simulink model "model_in_the_loop"  (R2017a)
settings: Solver=VariableStepAuto  StartTime=0.0  StopTime=10.0  RelTol=1e-3
values from neighbouring files (symbols this model uses):
  a = 31    [fun_h1.m]    (also in fun_h2.m; fun_h3.m; identyfikacja_sqrt_h1.m; lqr_indentyfikacja.m)
  b = 46.5    [fun_h2.m]    (also in identyfikacja_sqrt_h1.m = [(C1_0+delta_C1_0); (C1_0-delta_C1_0); (D1_0+delta_D1_0); (-; identyfikacja_sqrt_h2.m = [(C2_0+delta_C2_0); (C2_0-delta_C2_0); (D2_0+delta_D2_0); (-; identyfikacja_sqrt_h3.m = [(C3_0+delta_C3_0); (C3_0-delta_C3_0); (D3_0+delta_D3_0); (-; lqr_indentyfikacja.m)
  c = 10    [fun_h2.m]    (also in lqr_indentyfikacja.m; run_model.m)
  C1max = 36.9    [lqr_indentyfikacja.m]    (also in run_model.m)
  C2max = 33.91    [lqr_indentyfikacja.m]    (also in run_model.m)
  C3max = 36    [lqr_indentyfikacja.m]    (also in run_model.m)
  D1 = teta(2)    [fun_h1.m]    (also in lqr_indentyfikacja.m = 3.5673; run_model.m = 3.5673)
  D2 = teta(2)    [fun_h2.m]    (also in lqr_indentyfikacja.m = 2.8498; run_model.m = 2.8498)
  D3 = teta(2)    [fun_h3.m]    (also in lqr_indentyfikacja.m = 2.882; run_model.m = 2.882)
  gC1 = 1    [lqr_indentyfikacja.m]    (also in run_model.m)
  gC2 = 1    [lqr_indentyfikacja.m]    (also in run_model.m)
  gC3 = 1    [lqr_indentyfikacja.m]    (also in run_model.m)
  H10 = teta(4)    [fun_h1.m]    (also in lqr_indentyfikacja.m = 11.9703; run_model.m = 11.9703)
  H1OUT = ((C2*(r+D2)^p2)/C1)^2    (= 11.9703137378)    [lqr_indentyfikacja.m]
  H20 = teta(4)    [fun_h2.m]    (also in lqr_indentyfikacja.m = 15; run_model.m = 15)
  H2OUT = r    (= 15)    [lqr_indentyfikacja.m]
  H30 = teta(4)    [fun_h3.m]    (also in lqr_indentyfikacja.m = 12.5763; run_model.m = 12.5763)
  H3OUT = ((C2*(r+D2)^p2)/C3)^2    (= 12.5763108708)    [lqr_indentyfikacja.m]
  Hmax = 40    [lqr_indentyfikacja.m]    (also in run_model.m)
  p1 = teta(3)    [fun_h1.m]    (also in lqr_indentyfikacja.m = 0.41; run_model.m = 0.41)
  p2 = teta(3)    [fun_h2.m]    (also in lqr_indentyfikacja.m = 0.46; run_model.m = 0.46)
  p3 = teta(3)    [fun_h3.m]    (also in lqr_indentyfikacja.m = 0.37; run_model.m = 0.37)
  R = 20    [lqr_indentyfikacja.m]    (also in run_model.m = 39)
  w = 5    [fun_h1.m]    (also in fun_h2.m; fun_h3.m; lqr_indentyfikacja.m; run_model.m)
undefined symbols (not defined in the file or in its folder): K
settings Model: Creator=thepi  LastModifiedBy=thepi

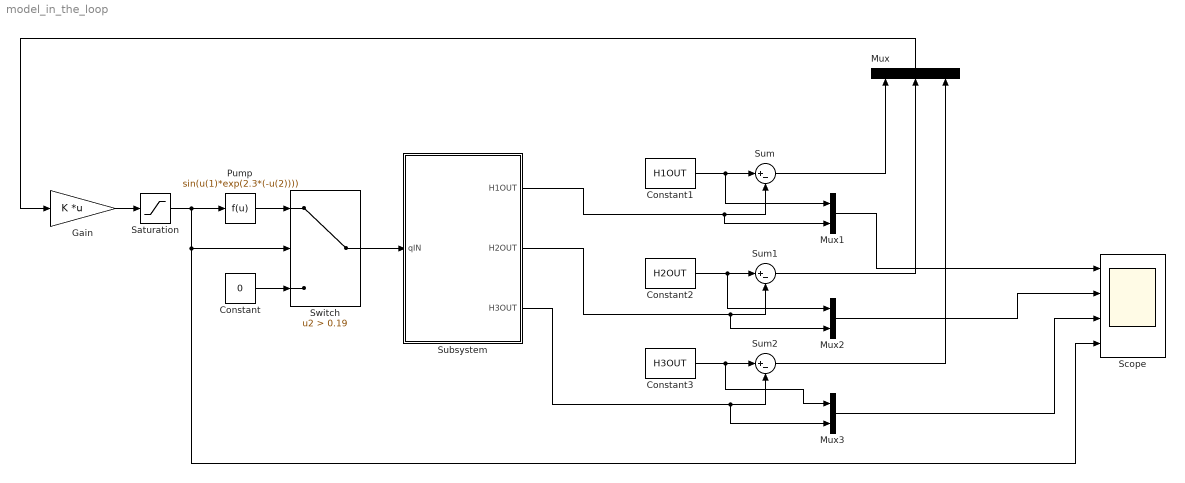
== system model_in_the_loop ==
  Constant : Constant  Value=0
  Constant1 : Constant  Value=H1OUT
  Constant2 : Constant  Value=H2OUT
  Constant3 : Constant  Value=H3OUT
  Gain : Gain  Gain=K  Multiplication=Matrix(K*u) (u vector)
  Mux : Mux  Inputs=3
  Mux1 : Mux  Inputs=2
  Mux2 : Mux  Inputs=2
  Mux3 : Mux  Inputs=2
  Pump : Fcn  Expr=sin(u(1)*exp(2.3*(-u(2))))
  Saturation : Saturate  UpperLimit=1  LowerLimit=0
  Scope : Scope  NumInputPorts=4
  Subsystem : Subsystem
  Sum : Sum  Inputs=|+-
  Sum1 : Sum  Inputs=|+-
  Sum2 : Sum  Inputs=|+-
  Switch : Switch  Criteria=u2 > Threshold  Threshold=0.19
  wires:
  Switch/1 -> Subsystem/1(qIN)
  Gain/1 -> Saturation/1
  Saturation/1 -> Scope/4, Switch/2, Pump/1
  Pump/1 -> Switch/1
  Constant/1 -> Switch/3
  Constant1/1 -> Mux1/1, Sum/1
  Constant3/1 -> Mux3/1, Sum2/1
  Constant2/1 -> Mux2/1, Sum1/1
  Sum/1 -> Mux/1
  Sum1/1 -> Mux/2
  Sum2/1 -> Mux/3
  Subsystem/1(H1OUT) -> Mux1/2, Sum/2
  Subsystem/2(H2OUT) -> Mux2/2, Sum1/2
  Subsystem/3(H3OUT) -> Mux3/2, Sum2/2
  Mux/1 -> Gain/1
  Mux1/1 -> Scope/1
  Mux2/1 -> Scope/2
  Mux3/1 -> Scope/3

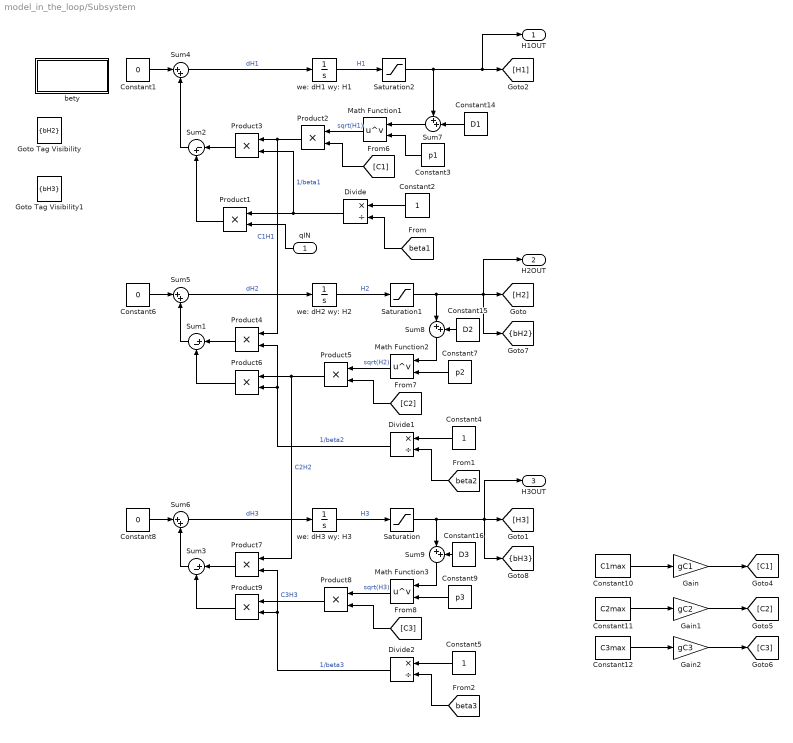
== system model_in_the_loop/Subsystem ==
  qIN : Inport
  Constant1 : Constant  Value=0
  Constant10 : Constant  Value=C1max
  Constant11 : Constant  Value=C2max
  Constant12 : Constant  Value=C3max
  Constant14 : Constant  Value=D1
  Constant15 : Constant  Value=D2
  Constant16 : Constant  Value=D3
  Constant2 : Constant
  Constant3 : Constant  Value=p1
  Constant4 : Constant
  Constant5 : Constant
  Constant6 : Constant  Value=0
  Constant7 : Constant  Value=p2
  Constant8 : Constant  Value=0
  Constant9 : Constant  Value=p3
  Divide : Product  Inputs=*/
  Divide1 : Product  Inputs=*/
  Divide2 : Product  Inputs=*/
  Gain : Gain  Gain=gC1
  Gain1 : Gain  Gain=gC2
  Gain2 : Gain  Gain=gC3
  Goto Tag Visibility : GotoTagVisibility  GotoTag=bH2
  Goto Tag Visibility1 : GotoTagVisibility  GotoTag=bH3
  Math Function1 : Math  Operator=pow  SaturateOnIntegerOverflow=on
  Math Function2 : Math  Operator=pow  SaturateOnIntegerOverflow=on
  Math Function3 : Math  Operator=pow  SaturateOnIntegerOverflow=on
  Product{1..9} (9 alike) : Product
  Saturation : Saturate  UpperLimit=R  LowerLimit=0
  Saturation1 : Saturate  UpperLimit=Hmax  LowerLimit=0
  Saturation2 : Saturate  UpperLimit=Hmax  LowerLimit=0
  Sum1 : Sum  Inputs=|+-
  Sum2 : Sum  Inputs=|-+
  Sum3 : Sum  Inputs=|+-
  Sum{4..6,8..9} (5 alike) : Sum  Inputs=|++
  Sum7 : Sum  Inputs=++|
  bety : Subsystem
  "we: dH1 wy: H1 " : Integrator  InitialCondition=H10  UpperSaturationLimit=40  LowerSaturationLimit=0
  we: dH2 wy: H2 : Integrator  InitialCondition=H20  UpperSaturationLimit=40  LowerSaturationLimit=0
  we: dH3 wy: H3 : Integrator  InitialCondition=H30  UpperSaturationLimit=40  LowerSaturationLimit=0
  H1OUT : Outport
  H2OUT : Outport  Port=2
  H3OUT : Outport  Port=3
  tag scope: bH2=scoped, bH3=scoped
  wires:
  [C1] -> Product2/2
  Constant4/1 -> Divide1/1
  Sum9/1 -> Math Function3/1
  Sum5/1 -> we: dH2 wy: H2/1  "dH2"
  [beta2] -> Divide1/2
  "we: dH1 wy: H1 "/1 -> Saturation2/1  "H1"
  Math Function2/1 -> Product5/1  "sqrt(H2)"
  Product4/1 -> Sum1/1
  Sum8/1 -> Math Function2/1
  Product2/1 -> Product4/1, Product3/1  "C1H1"
  we: dH2 wy: H2/1 -> Saturation1/1  "H2"
  Constant9/1 -> Math Function3/2
  Constant2/1 -> Divide/1
  Constant7/1 -> Math Function2/2
  qIN/1 -> Product1/2
  Saturation/1 -> Sum9/1, H3OUT/1, [bH3], [H3]
  Gain1/1 -> [C2]
  Sum6/1 -> we: dH3 wy: H3/1  "dH3"
  Constant8/1 -> Sum6/1
  Saturation1/1 -> Sum8/1, H2OUT/1, [bH2], [H2]
  Math Function1/1 -> Product2/1  "sqrt(H1)"
  Product1/1 -> Sum2/2
  Sum2/1 -> Sum4/2
  Gain2/1 -> [C3]
  Sum4/1 -> "we: dH1 wy: H1 "/1  "dH1"
  [beta1] -> Divide/2
  Constant6/1 -> Sum5/1
  Constant1/1 -> Sum4/1
  Constant16/1 -> Sum9/2
  [C2] -> Product5/2
  Divide2/1 -> Product7/2, Product9/2  "1/beta3"
  Sum3/1 -> Sum6/2
  Constant14/1 -> Sum7/2
  Divide1/1 -> Product6/2, Product4/2  "1/beta2"
  we: dH3 wy: H3/1 -> Saturation/1  "H3"
  Product7/1 -> Sum3/1
  Product8/1 -> Product9/1  "C3H3"
  Constant5/1 -> Divide2/1
  Product9/1 -> Sum3/2
  Divide/1 -> Product3/2, Product1/1  "1/beta1"
  Saturation2/1 -> Sum7/1, H1OUT/1, [H1]
  Constant12/1 -> Gain2/1
  [beta3] -> Divide2/2
  Sum1/1 -> Sum5/2
  Product5/1 -> Product7/1, Product6/1  "C2H2"
  Constant11/1 -> Gain1/1
  Product6/1 -> Sum1/2
  Math Function3/1 -> Product8/1  "sqrt(H3)"
  Constant10/1 -> Gain/1
  Constant15/1 -> Sum8/2
  Product3/1 -> Sum2/1
  Sum7/1 -> Math Function1/1
  Constant3/1 -> Math Function1/2
  [C3] -> Product8/2
  Gain/1 -> [C1]

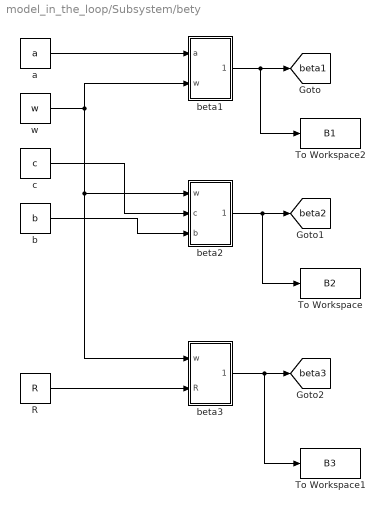
== system model_in_the_loop/Subsystem/bety ==
  R : Constant  Value=R
  To Workspace : ToWorkspace  VariableName=B2  SampleTime=-1
      settings: Save2DSignal=2-D array (concatenate along first dimension)
  To Workspace1 : ToWorkspace  VariableName=B3  SampleTime=-1
      settings: Save2DSignal=2-D array (concatenate along first dimension)
  To Workspace2 : ToWorkspace  VariableName=B1  SampleTime=-1
      settings: Save2DSignal=2-D array (concatenate along first dimension)
  a : Constant  Value=a
  b : Constant  Value=b
  beta1 : Subsystem
  "beta2 " : Subsystem
  beta3 : Subsystem
  c : Constant  Value=c
  w : Constant  Value=w
  tag scope: beta1=global, beta2=global, beta3=global
  wires:
  w/1 -> beta3/1(w), "beta2 "/1(w), beta1/2(w)
  a/1 -> beta1/1(a)
  beta1/1(Out1) -> To Workspace2/1, [beta1]
  c/1 -> "beta2 "/2(c)
  b/1 -> "beta2 "/3(b)
  R/1 -> beta3/2(R)
  "beta2 "/1(Out1) -> To Workspace/1, [beta2]
  beta3/1(Out1) -> To Workspace1/1, [beta3]

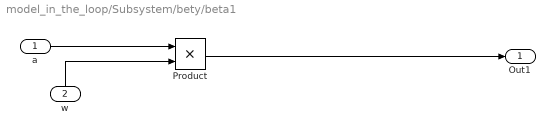
== system model_in_the_loop/Subsystem/bety/beta1 ==
  a : Inport
  w : Inport  Port=2
  Product : Product
  Out1 : Outport
  wires:
  Product/1 -> Out1/1
  a/1 -> Product/1
  w/1 -> Product/2

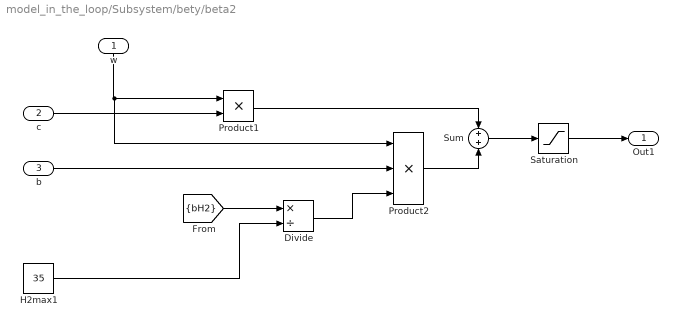
== system model_in_the_loop/Subsystem/bety/beta2  ==
  w : Inport
  c : Inport  Port=2
  b : Inport  Port=3
  Divide : Product  Inputs=*/
  H2max1 : Constant  Value=35
  Product1 : Product
  Product2 : Product  Inputs=3
  Saturation : Saturate  UpperLimit=w*(c+b)  LowerLimit=w*c
  Sum : Sum  Inputs=+|+
  Out1 : Outport
  wires:
  b/1 -> Product2/2
  Divide/1 -> Product2/3
  w/1 -> Product2/1, Product1/1
  Product2/1 -> Sum/2
  c/1 -> Product1/2
  [bH2] -> Divide/1
  H2max1/1 -> Divide/2
  Product1/1 -> Sum/1
  Sum/1 -> Saturation/1
  Saturation/1 -> Out1/1

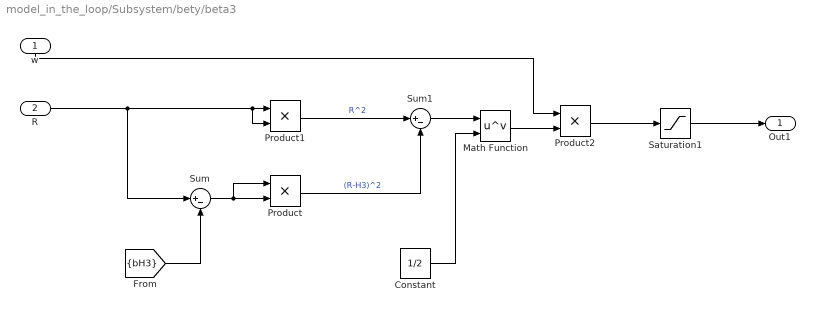
== system model_in_the_loop/Subsystem/bety/beta3 ==
  w : Inport
  R : Inport  Port=2
  Constant : Constant  Value=1/2
  Math Function : Math  Operator=pow  SaturateOnIntegerOverflow=on
  Product : Product
  Product1 : Product
  Product2 : Product
  Saturation1 : Saturate  UpperLimit=R*w  LowerLimit=0.001
  Sum : Sum  Inputs=|+-
  Sum1 : Sum  Inputs=|+-
  Out1 : Outport
  wires:
  R/1 -> Sum/1, Product1/2, Product1/1
  w/1 -> Product2/1
  Sum/1 -> Product/1, Product/2
  Sum1/1 -> Math Function/1
  Product/1 -> Sum1/2  "(R-H3)^2"
  Product1/1 -> Sum1/1  "R^2"
  Constant/1 -> Math Function/2
  Math Function/1 -> Product2/2
  [bH3] -> Sum/2
  Product2/1 -> Saturation1/1
  Saturation1/1 -> Out1/1
